simulink model "wmr_cmd_vel_subscriber"  (R2018b)
settings: Solver=VariableStepAuto  StartTime=0.0  StopTime=10  RelTol=1e-3
undefined symbols (not defined in the file or in its folder): Angular, Linear
libraries: robotlib x3
settings Model: Creator=robot  LastModifiedBy=robot

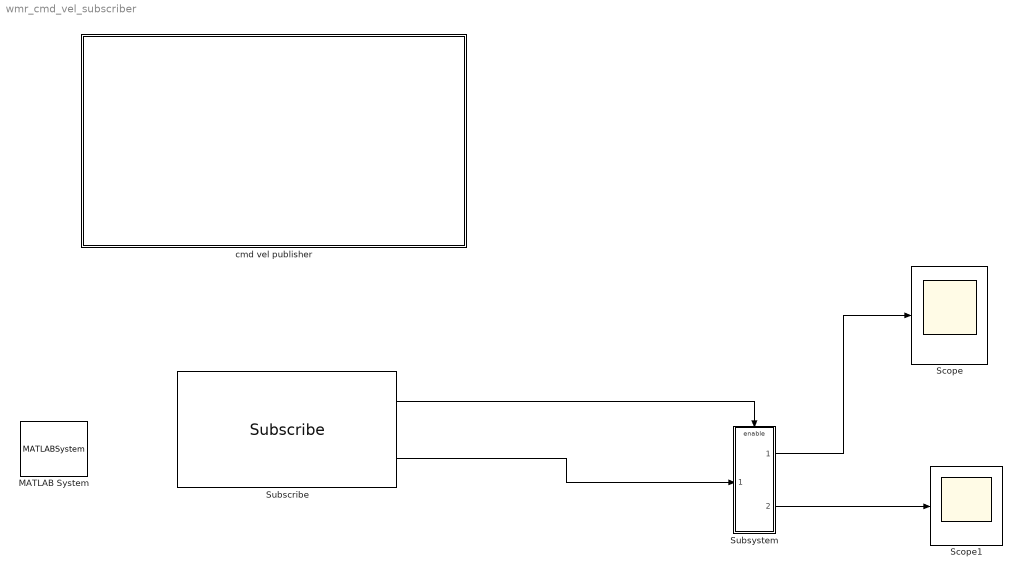
== system wmr_cmd_vel_subscriber ==
  MATLAB System : MATLABSystem  System=ros_rate  RATE=[0.5]  SimulateUsing=Code generation
      mask Type: ros_rate
      mask Display: disp('ros_rate');
  Scope : Scope
  Scope1 : Scope
  Subscribe : robotlib/Subscribe  topicSource=Select from ROS network  topic=/wmr_robot/odometry  messageType=nav_msgs/Odometry  sampleTime=-1  messageQueueLength=1
      settings: SourceProductBaseCode=RO
  Subsystem : Subsystem
  "cmd vel publisher " : Subsystem
  wires:
  Subscribe/2 -> Subsystem/1(In1)
  Subsystem/1(Out1) -> Scope/1
  Subsystem/2(Out2) -> Scope1/1
  Subscribe/1 -> Subsystem/Enable

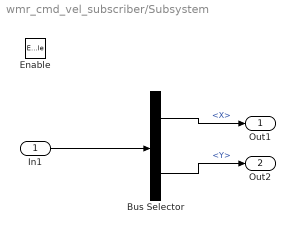
== system wmr_cmd_vel_subscriber/Subsystem ==
  In1 : Inport
  Enable : EnablePort
  Bus Selector : BusSelector  OutputSignals=Pose.Pose.Position.X,Pose.Pose.Position.Y
  Out1 : Outport
  Out2 : Outport  Port=2
  wires:
  Bus Selector/1 -> Out1/1  "<X>"
  In1/1 -> Bus Selector/1
  Bus Selector/2 -> Out2/1  "<Y>"

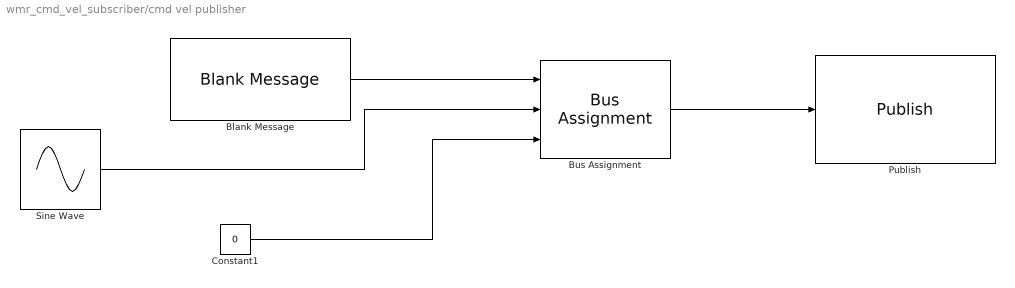
== system wmr_cmd_vel_subscriber/cmd vel publisher  ==
  Blank Message : robotlib/Blank Message  messageClass=Message  entityType=geometry_msgs/Twist  messageType=geometry_msgs/Twist  SampleTime=inf
      settings: SourceProductBaseCode=RO
  Bus Assignment : BusAssignment  AssignedSignals=Linear.X,Angular.Z
  Constant1 : Constant  Value=0
  Publish : robotlib/Publish  topicSource=Select from ROS network  topic=/cmd_vel  messageType=geometry_msgs/Twist  messageQueueLength=1
      settings: SourceProductBaseCode=RO
  Sine Wave : Sin  SampleTime=0
  wires:
  Sine Wave/1 -> Bus Assignment/2
  Bus Assignment/1 -> Publish/1
  Blank Message/1 -> Bus Assignment/1
  Constant1/1 -> Bus Assignment/3
